simulink model "Model_ukl_sprezystego"  (R2017b)
settings: Solver=ode1  StartTime=0.0  StopTime=9  FixedStep=0.0001  RelTol=1e-3
values from neighbouring files (symbols this model uses):
  Ki = T1/(T2*Tc)    (= 384.615384615)    [Dane_sprezyste.m]
  Kms = (((zeta^2*4*T1)/T2)-1)    (= 0.96)    [Dane_sprezyste.m]
  Kp = 4*T1*(sqrt((1+Kms)/(4*T1*Tc)))    [Dane_sprezyste.m]
  T1 = 0.203    [Dane_sprezyste.m]
  T2 = 0.203    [Dane_sprezyste.m]
  Tc = 0.0026    [Dane_sprezyste.m]
  Te = 0.0001    [Dane_sprezyste.m]
undefined symbols (not defined in the file or in its folder): sigbuilder_block
settings Model: Creator=kamil  LastModifiedBy=kamil

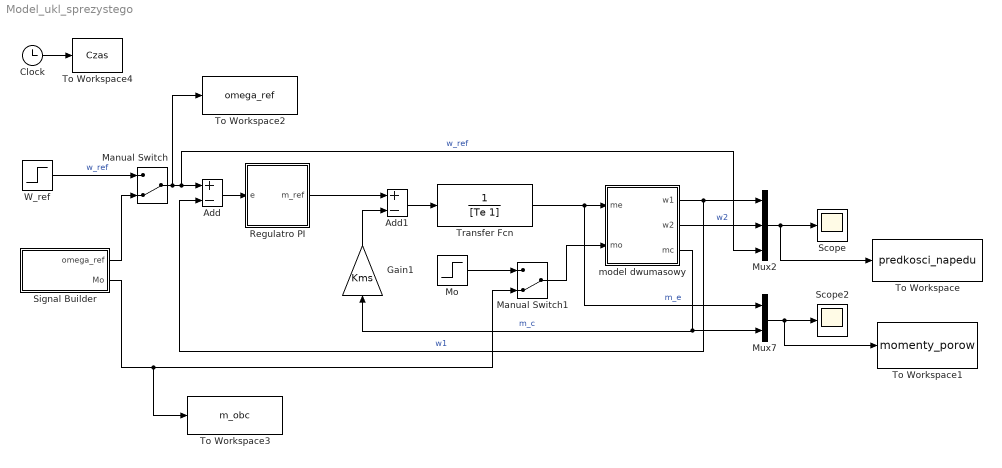
== system Model_ukl_sprezystego ==
  Add : Sum  Inputs=+-
  Add1 : Sum  Inputs=+-
  Clock : Clock
  Gain1 : Gain  Gain=Kms
  Manual Switch : ManualSwitch  CurrentSetting=0
  Manual Switch1 : ManualSwitch  CurrentSetting=0
  Mo : Step  Time=2  After=0.25  SampleTime=0
  Mux2 : Mux  Inputs=3
  Mux7 : Mux  Inputs=2
  Regulatro PI : Subsystem
  Scope : Scope
  Scope2 : Scope
  Signal Builder : Subsystem  Tag=STV Subsys  LoadFcn=sigbuilder_block('load');  StartFcn=sigbuilder_block('start');  StopFcn=sigbuilder_block('stop');  ClipboardFcn=sigbuilder_block('clipboard');  mask(Sigbuilder block){tuvar=[0:10]}
      mask help: Simulink:masks:SigbuilderBlock_MD
      mask init:
      | if ~strcmp(get_param(bdroot(gcbh),'SimulationStatus'),'stopped') tuvar = sigbuilder_block('maskInit'); end
      settings: CopyFcn=sigbuilder_block('copy');  DeleteFcn=sigbuilder_block('delete');  ModelCloseFcn=sigbuilder_block('modelClose');  PreSaveFcn=sigbuilder_block('preSave');  PauseFcn=sigbuilder_block('pause');  ContinueFcn=sigbuilder_block('continue');  NameChangeFcn=sigbuilder_block('namechange');  OpenFcn=sigbuilder_block('open',[217.2 110.4 550.8 400.2 ]);  CloseFcn=sigbuilder_block('close');
      mask Display: plot(0, 0, 100, 100,[2, 2, 32, 32, 2], [68, 8, 8, 68, 68],[32, 2], [38, 38], [32, 19, 2],[53, 60, 44], [32, 17, 17, 2],[16, 16, 31, 31]);txt = getActiveGroup(gcbh);text(2, 100, txt,'verticalAlignment', 'top');
  To Workspace : ToWorkspace  VariableName=predkosci_napedu  SampleTime=-1
  To Workspace1 : ToWorkspace  VariableName=momenty_porow  SampleTime=-1
  To Workspace2 : ToWorkspace  VariableName=omega_ref  SampleTime=-1
  To Workspace3 : ToWorkspace  VariableName=m_obc  SampleTime=-1
  To Workspace4 : ToWorkspace  VariableName=Czas  SampleTime=-1
  Transfer Fcn : TransferFcn  Denominator=[Te 1]
  W_ref : Step  Time=0.5  After=0.25  SampleTime=0
  "model dwumasowy " : Subsystem
  wires:
  Mux2/1 -> To Workspace/1, Scope/1
  "model dwumasowy "/3(mc) -> Mux7/2, Gain1/1  "m_c"
  "model dwumasowy "/2(w2) -> Mux2/2  "w2"
  Add/1 -> Regulatro PI/1(e)
  Transfer Fcn/1 -> Mux7/1, "model dwumasowy "/1(me)  "m_e"
  "model dwumasowy "/1(w1) -> Mux2/1, Add/2  "w1"
  Mux7/1 -> To Workspace1/1, Scope2/1
  Add1/1 -> Transfer Fcn/1
  Regulatro PI/1(m_ref) -> Add1/1
  Gain1/1 -> Add1/2
  Manual Switch/1 -> To Workspace2/1, Add/1, Mux2/3  "w_ref"
  W_ref/1 -> Manual Switch/1  "w_ref"
  Signal Builder/1(omega_ref) -> Manual Switch/2
  Manual Switch1/1 -> "model dwumasowy "/2(mo)
  Mo/1 -> Manual Switch1/1
  Signal Builder/2(Mo) -> To Workspace3/1, Manual Switch1/2
  Clock/1 -> To Workspace4/1

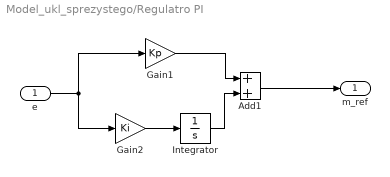
== system Model_ukl_sprezystego/Regulatro PI ==
  e : Inport
  Add1 : Sum
  Gain1 : Gain  Gain=Kp
  Gain2 : Gain  Gain=Ki
  Integrator : Integrator
  m_ref : Outport
  wires:
  Gain1/1 -> Add1/1
  Add1/1 -> m_ref/1
  e/1 -> Gain2/1, Gain1/1
  Gain2/1 -> Integrator/1
  Integrator/1 -> Add1/2

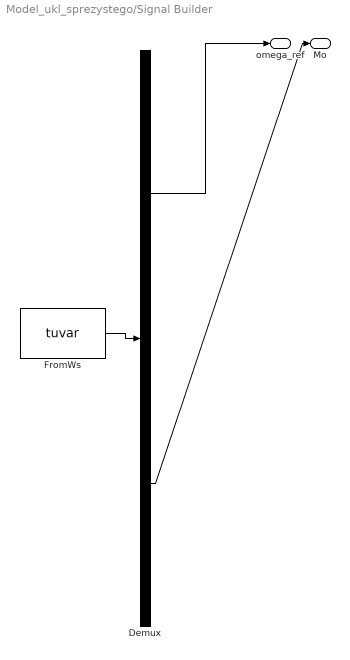
== system Model_ukl_sprezystego/Signal Builder ==
  Demux : Demux  Tag=STV Demux  Outputs=2
  FromWs : FromWorkspace  Tag=STV FromWs  VariableName=tuvar  SampleTime=0
      SigBuilderData=|
      | common.afterFinalStr = 'Extrapolate'
      | common.sampleTime = 0
      | dataSet.timeRange = [0 10]
      | dataSet.name = 'Group 1'
      | sbobj.Groups.Name = 'Group 1'
      | sbobj.Groups.Signals(1).Name = 'omega_ref'
      | sbobj.Groups.Signals(1).XData = [0 1 1 2 2 3 3 4 4 5 6.5 7.5 7.5 8.5 8.5 10]
      | sbobj.Groups.Signals(1).YData = [0 0 0.2 0.2 0.45 0.45 0.65 0.65 1 1 -0.1 -0.1 -0.35 -0.35 -0.5 -0.5]
      | sbobj.Groups.Signals(2).Name = 'Mo'
      | sbobj.Groups.Signals(2).XData = [0 0.4 0.4 0.6 0.6 1.4 1.4 1.6 1.6 2.4 2.4 2.6 2.6 3.4 3.4 3.58 3.58 4.4 4.4 4.6 4.6 6.8 6.8 7 7 7.9 7.9 8.1 8.1 9.2 9.2 9.4 9.4 10]
      | sbobj.Groups.Signals(2).YData = [0 0 1 1 0 0 1 1 0 0 1 1 0 0 1 1 0 0.00281915973209 1.01 1.01 0.00312522833367 0.00668033285975 1.01 1.01 0.00696285772275 0.00750436371017 1 1 0.00778688857317 0.00832839456058 1 1 0.00861091942358 0.01]
      | sbobj.Groups.TimeRange = [0 10]
  omega_ref : Outport  Tag=STV Outport
  Mo : Outport  Tag=STV Outport  Port=2
  wires:
  Demux/1 -> omega_ref/1
  FromWs/1 -> Demux/1
  Demux/2 -> Mo/1

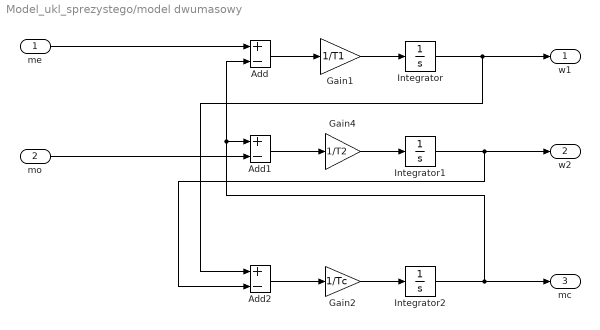
== system Model_ukl_sprezystego/model dwumasowy  ==
  me : Inport
  mo : Inport  Port=2
  Add : Sum  Inputs=+-
  Add1 : Sum  Inputs=+-
  Add2 : Sum  Inputs=+-
  Gain1 : Gain  Gain=1/T1
  Gain2 : Gain  Gain=1/Tc
  Gain4 : Gain  Gain=1/T2
  Integrator : Integrator
  Integrator1 : Integrator
  Integrator2 : Integrator
  w1 : Outport
  w2 : Outport  Port=2
  mc : Outport  Port=3
  wires:
  Integrator/1 -> w1/1, Add2/1
  Integrator2/1 -> mc/1, Add/2, Add1/1
  Integrator1/1 -> w2/1, Add2/2
  Add/1 -> Gain1/1
  Gain1/1 -> Integrator/1
  Add1/1 -> Gain4/1
  Gain4/1 -> Integrator1/1
  Add2/1 -> Gain2/1
  Gain2/1 -> Integrator2/1
  mo/1 -> Add1/2
  me/1 -> Add/1
